simulink model "finalSimscapeModel"  (R2021b)
settings: Solver=FixedStepAuto  StartTime=0.0  StopTime=30+2*time_sequence(end)  FixedStep=0.05  RelTol=1e-3
libraries: nesl_utility x25, sm_lib x16, vrlib x6
settings Model: Creator=mukes  LastModifiedBy=mukes
settings ExplorerConfigSet: InternalSimMechanicsExplorerSettings="<ExplorerConfiguration><canonicalview>default</canonicalview><AnimationSetting><BasePlaybackSpeed>1.0</BasePlaybackSpeed><PlaybackSpeedFactor>1.0</PlaybackSpeedFactor></AnimationSetting><TilePanel><TileInfo><Tiles Columns=\"1\" Count=\"1\" Rows=\"1\"><Column Weight=\"1\"/><Row Weight=\"1\"/><Tile Height=\"1\" Width=\"1\" X=\"0\" Y=\"0\"/></Tiles></TileInfo><SceneInfo><SceneViewer><BGColor><R>0.60000002384185791</R><G>0.60000002384185791</G><B>0.60000002384185791</B></BGColor><Camera><DoPerspective>on</DoPerspective><Position><X>0.947420253079612085</X><Y>-0.0616353411456797562</Y><Z>0.809347594742444554</Z></Position><Center><X>-2.25255068230077837</X><Y>-0.872881532072153465</Y><Z>0.964544977754672184</Z></Center><Up><X>0.118811010900315428</X><Y>-0.286795567538067564</Y><Z>0.950595732227618839</Z></Up><ViewLimDist>1</ViewLimDist><YLim>0.466307658154998583</YLim><XLim>0.755157212465178973</XLim></Camera></SceneViewer></SceneInfo></TilePanel><MechEditorPanel><Cameras><Camera><Id>Camera1</Id><Value><Name>Camera1</Name><NativeCamera><PositionKeyframeSet><Keyframe><Time>50</Time><Value><X>2.03308088006994</X><Y>0.9365322772522765</Y><Z>2.5154667404724962</Z></Value></Keyframe></PositionKeyframeSet><CenterKeyframeSet><Keyframe><Time>50</Time><Value><X>-0.070008809160188701</X><Y>-0.63944287284674839</Y><Z>1.2349132743696094</Z></Value></Keyframe></CenterKeyframeSet><UpVectorKeyframeSet><Keyframe><Time>50</Time><Value><X>-0.43034741458034742</X><Y>-0.14909651685273262</Y><Z>0.89026475355727386</Z></Value></Keyframe></UpVectorKeyframeSet></NativeCamera></Value></Camera></Cameras><GfxPanelCameraMap><MapElement CameraMLId=\"Camera1\" GfxPanelIndex=\"0\"/></GfxPanelCameraMap><VideoCreator><PlaybackSpeedRatio>1.0</PlaybackSpeedRatio><FrameRate>30</FrameRate><VideoFormat>Motion JPEG AVI</VideoFormat><FrameSize>auto</FrameSize></VideoCreator></MechEditorPanel></ExplorerConfiguration>"

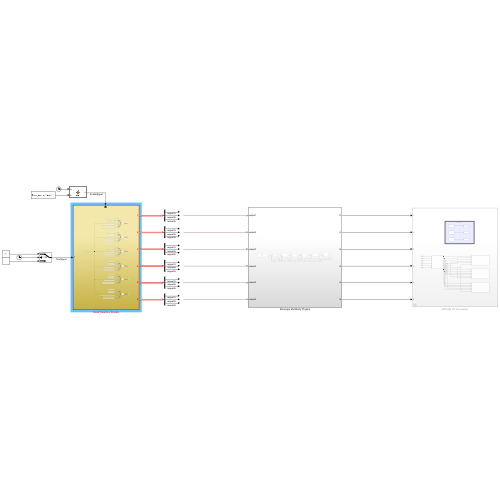
[thumbnail: Simulink's stored preview of the top-level diagram]
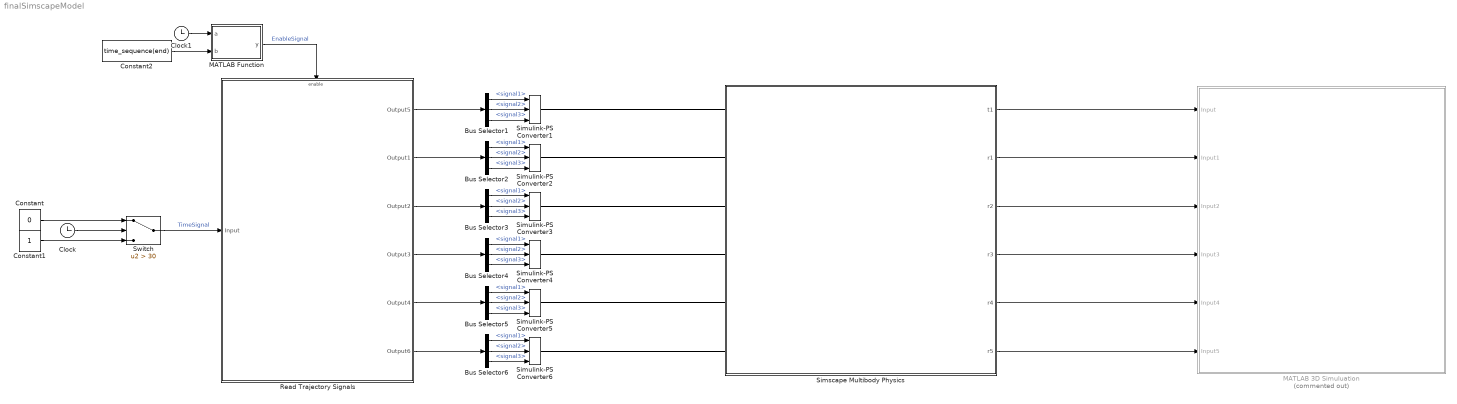
== system finalSimscapeModel ==
  Bus Selector{1..6} (6 alike) : BusSelector  OutputSignals=signal1,signal2,signal3
  Clock : Clock
  Clock1 : Clock
  Constant : Constant  Value=0
  Constant1 : Constant
  Constant2 : Constant  Value=time_sequence(end)
  MATLAB 3D Simuluation : Subsystem  Commented=on
  MATLAB Function : MATLAB Function  TreatAsAtomicUnit=on
  Read Trajectory Signals : Subsystem
  Simscape Multibody Physics : Subsystem
  Simulink-PS Converter{1..6} (6 alike) : nesl_utility/Simulink-PS Converter  PhysicalDomain=network_engine_domain  SubClassName=ps_input  LeftPortType=input  RightPortType=output  PseudoPeriodic=off  Frequencies=[]  NoiseDistribution=none  NoiseParameters=[]  Unit=1  AffineConversion=off  FilteringAndDerivatives=provide  SimscapeFilterOrder=1  InputFilterTimeConstant=0.001  UdotUserProvided=2
      settings: SourceProductBaseCode=PW,SS
  Switch : Switch  Criteria=u2 > Threshold  Threshold=30
  wires:
  Switch/1 -> Read Trajectory Signals/1(Input)  "TimeSignal"
  Constant/1 -> Switch/1
  Clock/1 -> Switch/2
  Constant1/1 -> Switch/3
  Bus Selector1/2 -> Simulink-PS Converter1/2  "<signal2>"
  Read Trajectory Signals/1(Output5) -> Bus Selector1/1
  Bus Selector1/3 -> Simulink-PS Converter1/3  "<signal3>"
  Bus Selector1/1 -> Simulink-PS Converter1/1  "<signal1>"
  Bus Selector2/2 -> Simulink-PS Converter2/2  "<signal2>"
  Read Trajectory Signals/2(Output1) -> Bus Selector2/1
  Bus Selector2/3 -> Simulink-PS Converter2/3  "<signal3>"
  Bus Selector2/1 -> Simulink-PS Converter2/1  "<signal1>"
  Bus Selector3/2 -> Simulink-PS Converter3/2  "<signal2>"
  Bus Selector3/1 -> Simulink-PS Converter3/1  "<signal1>"
  Bus Selector3/3 -> Simulink-PS Converter3/3  "<signal3>"
  Read Trajectory Signals/3(Output2) -> Bus Selector3/1
  Bus Selector4/2 -> Simulink-PS Converter4/2  "<signal2>"
  Bus Selector4/1 -> Simulink-PS Converter4/1  "<signal1>"
  Bus Selector4/3 -> Simulink-PS Converter4/3  "<signal3>"
  Read Trajectory Signals/4(Output3) -> Bus Selector4/1
  Bus Selector5/2 -> Simulink-PS Converter5/2  "<signal2>"
  Bus Selector5/1 -> Simulink-PS Converter5/1  "<signal1>"
  Bus Selector5/3 -> Simulink-PS Converter5/3  "<signal3>"
  Read Trajectory Signals/5(Output4) -> Bus Selector5/1
  Bus Selector6/2 -> Simulink-PS Converter6/2  "<signal2>"
  Bus Selector6/1 -> Simulink-PS Converter6/1  "<signal1>"
  Bus Selector6/3 -> Simulink-PS Converter6/3  "<signal3>"
  Read Trajectory Signals/6(Output6) -> Bus Selector6/1
  Clock1/1 -> MATLAB Function/1(a)
  Constant2/1 -> MATLAB Function/2(b)
  MATLAB Function/1(y) -> Read Trajectory Signals/Enable  "EnableSignal"
  Simscape Multibody Physics/1(t1) -> MATLAB 3D Simuluation/1(Input)
  Simscape Multibody Physics/2(r1) -> MATLAB 3D Simuluation/2(Input1)
  Simscape Multibody Physics/3(r2) -> MATLAB 3D Simuluation/3(Input2)
  Simscape Multibody Physics/4(r3) -> MATLAB 3D Simuluation/4(Input3)
  Simscape Multibody Physics/5(r4) -> MATLAB 3D Simuluation/5(Input4)
  Simscape Multibody Physics/6(r5) -> MATLAB 3D Simuluation/6(Input5)
  connections:
  Simulink-PS Converter1/RConn1 -- Simscape Multibody Physics/LConn1
  Simulink-PS Converter2/RConn1 -- Simscape Multibody Physics/LConn2
  Simulink-PS Converter3/RConn1 -- Simscape Multibody Physics/LConn3
  Simulink-PS Converter4/RConn1 -- Simscape Multibody Physics/LConn4
  Simulink-PS Converter5/RConn1 -- Simscape Multibody Physics/LConn5
  Simulink-PS Converter6/RConn1 -- Simscape Multibody Physics/LConn6

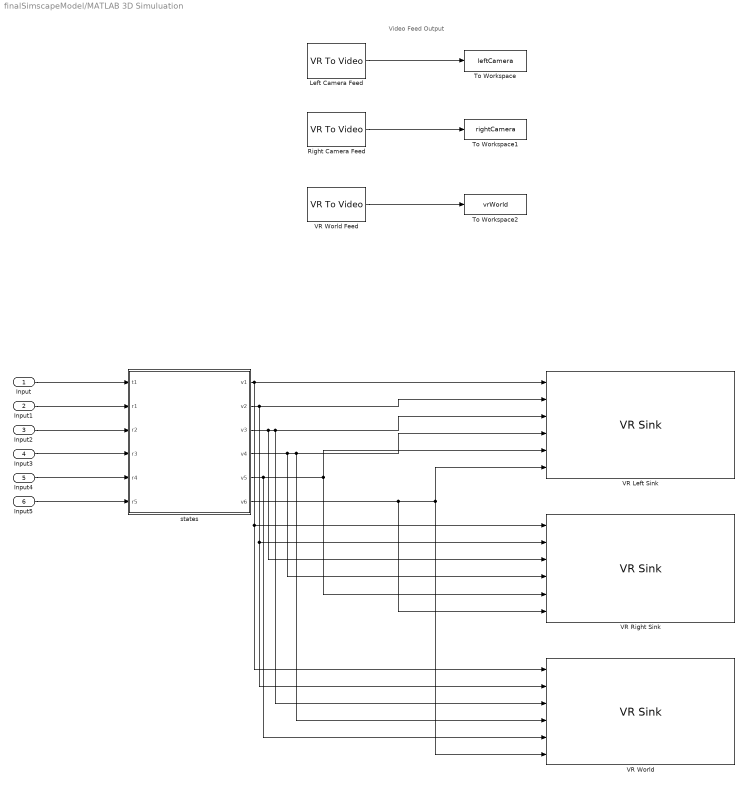
== system finalSimscapeModel/MATLAB 3D Simuluation ==
  note: Video Feed Output
  Input : Inport
  Input1 : Inport  Port=2
  Input2 : Inport  Port=3
  Input3 : Inport  Port=4
  Input4 : Inport  Port=5
  Input5 : Inport  Port=6
  Left Camera Feed : vrlib/VR To Video  InstantiateOnLoad=on  SampleTime=0.1  ViewEnable=on  RemoteChange=off  RemoteView=off  WorldFileName=jlr_world_final2_left.x3d  WorldDescription=Straight Road Strip - 2 Lanes  AutoView=off  VideoDimensions=[1080 1920]  AllowVariableSize=off
      settings: SourceProductBaseCode=SL
  Right Camera Feed : vrlib/VR To Video  InstantiateOnLoad=on  SampleTime=0.1  ViewEnable=on  RemoteChange=off  RemoteView=off  WorldFileName=jlr_world_final2_right.x3d  WorldDescription=Straight Road Strip - 2 Lanes  AutoView=off  VideoDimensions=[1080 1920]  AllowVariableSize=off
      settings: SourceProductBaseCode=SL
  To Workspace : ToWorkspace  VariableName=leftCamera  SaveFormat=Timeseries  SampleTime=-1
  To Workspace1 : ToWorkspace  VariableName=rightCamera  SaveFormat=Timeseries  SampleTime=-1
  To Workspace2 : ToWorkspace  VariableName=vrWorld  SaveFormat=Timeseries  SampleTime=-1
  VR Left Sink : vrlib/VR Sink  InstantiateOnLoad=on  SampleTime=0.1  ViewEnable=on  RemoteChange=off  RemoteView=off  FieldsWritten=axis_Trans1.translation.3.1.1.double#axis_Rev1.rotation.4.1.1.double#axis_Rev2.rotation.4.1.1.double#axis_Rev3.rotation.4.1.1.double#axis_Rev4.rotation.4.1.1.double#axis_Rev5.rotation.4.1.1.double  WorldFileName=jlr_world_final2_left.x3d  WorldDescription=Straight Road Strip - 2 Lanes  AutoView=off  VideoDimensions=[]  AllowVariableSize=off
  VR Right Sink : vrlib/VR Sink  InstantiateOnLoad=on  SampleTime=0.1  ViewEnable=on  RemoteChange=off  RemoteView=off  FieldsWritten=axis_Trans1.translation.3.1.1.double#axis_Rev1.rotation.4.1.1.double#axis_Rev2.rotation.4.1.1.double#axis_Rev3.rotation.4.1.1.double#axis_Rev4.rotation.4.1.1.double#axis_Rev5.rotation.4.1.1.double  WorldFileName=jlr_world_final2_right.x3d  WorldDescription=Straight Road Strip - 2 Lanes  AutoView=off  VideoDimensions=[]  AllowVariableSize=off
  VR World : vrlib/VR Sink  InstantiateOnLoad=on  SampleTime=0.1  ViewEnable=on  RemoteChange=off  RemoteView=off  FieldsWritten=axis_Trans1.translation.3.1.1.double#axis_Rev1.rotation.4.1.1.double#axis_Rev2.rotation.4.1.1.double#axis_Rev3.rotation.4.1.1.double#axis_Rev4.rotation.4.1.1.double#axis_Rev5.rotation.4.1.1.double  WorldFileName=jlr_world_final2.x3d  WorldDescription=Straight Road Strip - 2 Lanes  AutoView=off  VideoDimensions=[]  AllowVariableSize=off
  VR World Feed : vrlib/VR To Video  InstantiateOnLoad=on  SampleTime=0.1  ViewEnable=on  RemoteChange=off  RemoteView=off  WorldFileName=jlr_world_final2.x3d  WorldDescription=Straight Road Strip - 2 Lanes  AutoView=off  VideoDimensions=[1080 1920]  AllowVariableSize=off
      settings: SourceProductBaseCode=SL
  states : MATLAB Function  TreatAsAtomicUnit=on
  wires:
  states/6(v6) -> VR World/6, VR Left Sink/6, VR Right Sink/6
  states/5(v5) -> VR Right Sink/5, VR Left Sink/5, VR World/5
  states/4(v4) -> VR World/4, VR Left Sink/4, VR Right Sink/4
  states/1(v1) -> VR Right Sink/1, VR World/1, VR Left Sink/1
  states/2(v2) -> VR World/2, VR Right Sink/2, VR Left Sink/2
  Input2/1 -> states/3(r2)
  states/3(v3) -> VR World/3, VR Left Sink/3, VR Right Sink/3
  Input4/1 -> states/5(r4)
  Input1/1 -> states/2(r1)
  Input5/1 -> states/6(r5)
  Input3/1 -> states/4(r3)
  Input/1 -> states/1(t1)
  Left Camera Feed/1 -> To Workspace/1
  Right Camera Feed/1 -> To Workspace1/1
  VR World Feed/1 -> To Workspace2/1

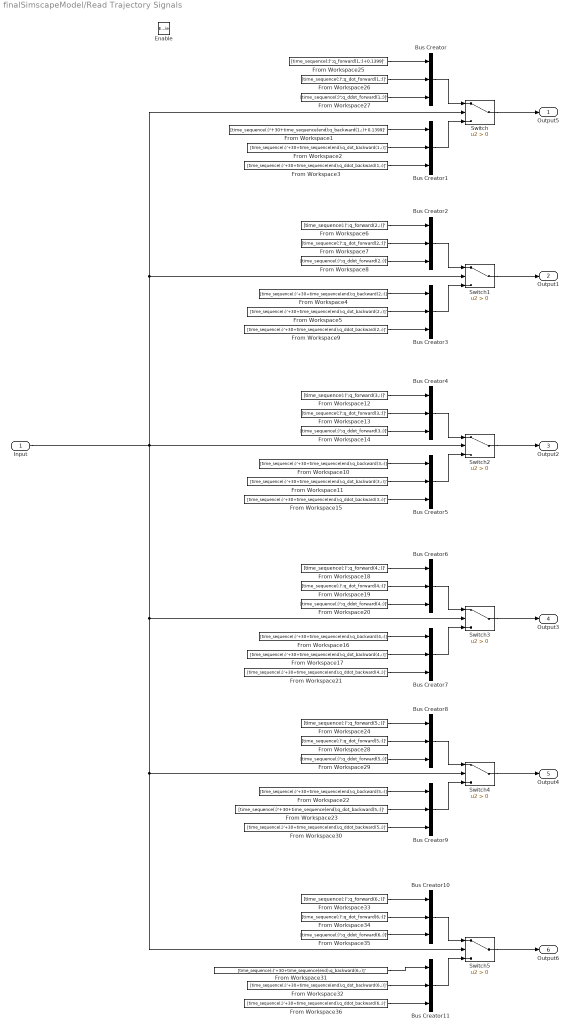
== system finalSimscapeModel/Read Trajectory Signals ==
  Input : Inport
  Enable : EnablePort
  Bus Creator{,1..11} (12 alike) : BusCreator  Inputs=3
  From Workspace1 : FromWorkspace  VariableName=[time_sequence(:)'+30+time_sequence(end);q_backward(1,:)+0.1399]'
  From Workspace10 : FromWorkspace  VariableName=[time_sequence(:)'+30+time_sequence(end);q_backward(3,:)]'
  From Workspace11 : FromWorkspace  VariableName=[time_sequence(:)'+30+time_sequence(end);q_dot_backward(3,:)]'
  From Workspace12 : FromWorkspace  VariableName=[time_sequence(:)';q_forward(3,:)]'
  From Workspace13 : FromWorkspace  VariableName=[time_sequence(:)';q_dot_forward(3,:)]'
  From Workspace14 : FromWorkspace  VariableName=[time_sequence(:)';q_ddot_forward(3,:)]'
  From Workspace15 : FromWorkspace  VariableName=[time_sequence(:)'+30+time_sequence(end);q_ddot_backward(3,:)]'
  From Workspace16 : FromWorkspace  VariableName=[time_sequence(:)'+30+time_sequence(end);q_backward(4,:)]'
  From Workspace17 : FromWorkspace  VariableName=[time_sequence(:)'+30+time_sequence(end);q_dot_backward(4,:)]'
  From Workspace18 : FromWorkspace  VariableName=[time_sequence(:)';q_forward(4,:)]'
  From Workspace19 : FromWorkspace  VariableName=[time_sequence(:)';q_dot_forward(4,:)]'
  From Workspace2 : FromWorkspace  VariableName=[time_sequence(:)'+30+time_sequence(end);q_dot_backward(1,:)]'
  From Workspace20 : FromWorkspace  VariableName=[time_sequence(:)';q_ddot_forward(4,:)]'
  From Workspace21 : FromWorkspace  VariableName=[time_sequence(:)'+30+time_sequence(end);q_ddot_backward(4,:)]'
  From Workspace22 : FromWorkspace  VariableName=[time_sequence(:)'+30+time_sequence(end);q_backward(5,:)]'
  From Workspace23 : FromWorkspace  VariableName=[time_sequence(:)'+30+time_sequence(end);q_dot_backward(5,:)]'
  From Workspace24 : FromWorkspace  VariableName=[time_sequence(:)';q_forward(5,:)]'
  From Workspace25 : FromWorkspace  VariableName=[time_sequence(:)';q_forward(1,:)+0.1399]'
  From Workspace26 : FromWorkspace  VariableName=[time_sequence(:)';q_dot_forward(1,:)]'
  From Workspace27 : FromWorkspace  VariableName=[time_sequence(:)';q_ddot_forward(1,:)]'
  From Workspace28 : FromWorkspace  VariableName=[time_sequence(:)';q_dot_forward(5,:)]'
  From Workspace29 : FromWorkspace  VariableName=[time_sequence(:)';q_ddot_forward(5,:)]'
  From Workspace3 : FromWorkspace  VariableName=[time_sequence(:)'+30+time_sequence(end);q_ddot_backward(1,:)]'
  From Workspace30 : FromWorkspace  VariableName=[time_sequence(:)'+30+time_sequence(end);q_ddot_backward(5,:)]'
  From Workspace31 : FromWorkspace  VariableName=[time_sequence(:)'+30+time_sequence(end);q_backward(6,:)]'
  From Workspace32 : FromWorkspace  VariableName=[time_sequence(:)'+30+time_sequence(end);q_dot_backward(6,:)]'
  From Workspace33 : FromWorkspace  VariableName=[time_sequence(:)';q_forward(6,:)]'
  From Workspace34 : FromWorkspace  VariableName=[time_sequence(:)';q_dot_forward(6,:)]'
  From Workspace35 : FromWorkspace  VariableName=[time_sequence(:)';q_ddot_forward(6,:)]'
  From Workspace36 : FromWorkspace  VariableName=[time_sequence(:)'+30+time_sequence(end);q_ddot_backward(6,:)]'
  From Workspace4 : FromWorkspace  VariableName=[time_sequence(:)'+30+time_sequence(end);q_backward(2,:)]'
  From Workspace5 : FromWorkspace  VariableName=[time_sequence(:)'+30+time_sequence(end);q_dot_backward(2,:)]'
  From Workspace6 : FromWorkspace  VariableName=[time_sequence(:)';q_forward(2,:)]'
  From Workspace7 : FromWorkspace  VariableName=[time_sequence(:)';q_dot_forward(2,:)]'
  From Workspace8 : FromWorkspace  VariableName=[time_sequence(:)';q_ddot_forward(2,:)]'
  From Workspace9 : FromWorkspace  VariableName=[time_sequence(:)'+30+time_sequence(end);q_ddot_backward(2,:)]'
  Switch{,1..5} (6 alike) : Switch  Criteria=u2 > Threshold
  Output5 : Outport
  Output1 : Outport  Port=2
  Output2 : Outport  Port=3
  Output3 : Outport  Port=4
  Output4 : Outport  Port=5
  Output6 : Outport  Port=6
  wires:
  From Workspace25/1 -> Bus Creator/1
  From Workspace26/1 -> Bus Creator/2
  From Workspace27/1 -> Bus Creator/3
  From Workspace1/1 -> Bus Creator1/1
  From Workspace3/1 -> Bus Creator1/3
  From Workspace2/1 -> Bus Creator1/2
  Bus Creator/1 -> Switch/1
  Bus Creator1/1 -> Switch/3
  Input/1 -> Switch1/2, Switch/2, Switch2/2, Switch5/2, Switch4/2, Switch3/2
  Switch/1 -> Output5/1
  Switch1/1 -> Output1/1
  From Workspace4/1 -> Bus Creator3/1
  Bus Creator3/1 -> Switch1/3
  From Workspace6/1 -> Bus Creator2/1
  From Workspace7/1 -> Bus Creator2/2
  Bus Creator2/1 -> Switch1/1
  From Workspace9/1 -> Bus Creator3/3
  From Workspace5/1 -> Bus Creator3/2
  From Workspace8/1 -> Bus Creator2/3
  Switch2/1 -> Output2/1
  From Workspace10/1 -> Bus Creator5/1
  Bus Creator5/1 -> Switch2/3
  From Workspace12/1 -> Bus Creator4/1
  From Workspace13/1 -> Bus Creator4/2
  Bus Creator4/1 -> Switch2/1
  From Workspace15/1 -> Bus Creator5/3
  From Workspace11/1 -> Bus Creator5/2
  From Workspace14/1 -> Bus Creator4/3
  Switch3/1 -> Output3/1
  From Workspace16/1 -> Bus Creator7/1
  Bus Creator7/1 -> Switch3/3
  From Workspace18/1 -> Bus Creator6/1
  From Workspace19/1 -> Bus Creator6/2
  Bus Creator6/1 -> Switch3/1
  From Workspace21/1 -> Bus Creator7/3
  From Workspace17/1 -> Bus Creator7/2
  From Workspace20/1 -> Bus Creator6/3
  Switch4/1 -> Output4/1
  From Workspace22/1 -> Bus Creator9/1
  Bus Creator9/1 -> Switch4/3
  From Workspace24/1 -> Bus Creator8/1
  From Workspace28/1 -> Bus Creator8/2
  Bus Creator8/1 -> Switch4/1
  From Workspace30/1 -> Bus Creator9/3
  From Workspace23/1 -> Bus Creator9/2
  From Workspace29/1 -> Bus Creator8/3
  Switch5/1 -> Output6/1
  From Workspace31/1 -> Bus Creator11/1
  Bus Creator11/1 -> Switch5/3
  From Workspace33/1 -> Bus Creator10/1
  From Workspace34/1 -> Bus Creator10/2
  Bus Creator10/1 -> Switch5/1
  From Workspace36/1 -> Bus Creator11/3
  From Workspace32/1 -> Bus Creator11/2
  From Workspace35/1 -> Bus Creator10/3

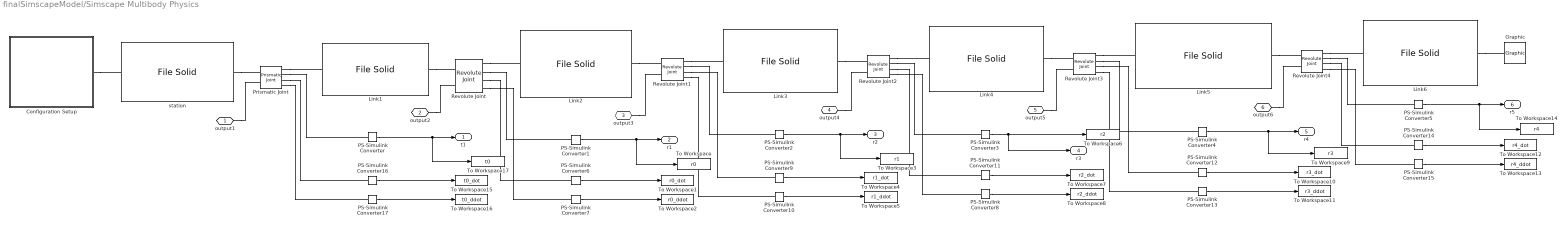
== system finalSimscapeModel/Simscape Multibody Physics ==
  Configuration Setup : Subsystem
  Graphic : sm_lib/Body Elements/Graphic  GraphicType=Marker  MarkerShape=Sphere  MarkerSize=10  GraphicVisPropType=SimpleVisualProperties  GraphicDiffuseColor=[1 0 0]  GraphicSpecularColor=[0.5 0.5 0.5 1.0]  GraphicAmbientColor=[0.15 0.15 0.15 1.0]  GraphicEmissiveColor=[0.0 0.0 0.0 1.0]  GraphicShininess=75  GraphicOpacity=1.0
  Link1 : sm_lib/Body Elements/File Solid  ExtGeomFileName=C:\Users\mukes\Downloads\Robot-Arm\Simscape Simulation\cadModels\Link1.STEP  UnitType=FromFile  ExtGeomFileUnits=m  StepReaderType=HEX  ExportConvexHullGeometry=off  InertiaType=CalculateFromGeometry  Mass=1  MassUnits=kg  CenterOfMass=[0 0 0]  CenterOfMassUnits=m  MomentsOfInertia=[1 1 1]  MomentsOfInertiaUnits=kg*m^2  ProductsOfInertia=[0 0 0]  ProductsOfInertiaUnits=kg*m^2  BasedOnType=Density  Density=1000  DensityUnits=kg/m^3  DoExposeReferenceFrame=off  SerializedFrames=<Frames><Frame><Id>Frame1</Id><Value><Name>prismaticJoint</Name><Origin><Source>GeometricFeature</Source><FeatureName>circular curve 1514</FeatureName></Origin><PrimaryAxis><DefinedDirection>+Z</DefinedDirection><Source>GeometricFeature</Source><SourceDirection>+Z</SourceDirection><FeatureName>circular curve 1514</FeatureName></PrimaryAxis><SecondaryAxis><DefinedDirection>+X</DefinedDirection><Source>GeometricFeature</Source><SourceDirection>+X</SourceDirection><FeatureName>segment 1580</FeatureName></SecondaryAxis></Value></Frame><Frame><Id>Frame2</Id><Value><Name>revoluteJoint</Name><Origin><Source>GeometricFeature</Source><FeatureName>circular curve 835</FeatureName></Origin><PrimaryAxis><DefinedDirection>-Z</DefinedDirection><Source>GeometricFeature</Source><SourceDirection>+Z</SourceDirection><FeatureName>circular curve 835</FeatureName></PrimaryAxis><SecondaryAxis><DefinedDirection>+X</DefinedDirection><Source>GeometricFeature</Source><SourceDirection>+X</SourceDirection><FeatureName>segment 1054</FeatureName></SecondaryAxis></Value></Frame></Frames>  GraphicType=FromGeometry  MarkerShape=Sphere  MarkerSize=10  GraphicVisPropType=SimpleVisualProperties  GraphicDiffuseColor=[0.5 0.5 0.5]  GraphicSpecularColor=[0.5 0.5 0.5 1.0]  GraphicAmbientColor=[0.15 0.15 0.15 1.0]  GraphicEmissiveColor=[0.0 0.0 0.0 1.0]  GraphicShininess=75  GraphicOpacity=1.0
  Link2 : sm_lib/Body Elements/File Solid  ExtGeomFileName=.\cadModels\Link2.STEP  UnitType=FromFile  ExtGeomFileUnits=m  StepReaderType=HEX  ExportConvexHullGeometry=off  InertiaType=CalculateFromGeometry  Mass=1  MassUnits=kg  CenterOfMass=[0 0 0]  CenterOfMassUnits=m  MomentsOfInertia=[1 1 1]  MomentsOfInertiaUnits=kg*m^2  ProductsOfInertia=[0 0 0]  ProductsOfInertiaUnits=kg*m^2  BasedOnType=Density  Density=1000  DensityUnits=kg/m^3  DoExposeReferenceFrame=off  SerializedFrames=<Frames><Frame><Id>Frame1</Id><Value><Name>revoluteJoint1</Name><Origin><Source>GeometricFeature</Source><FeatureName>circular curve 1127</FeatureName></Origin><PrimaryAxis><DefinedDirection>-Z</DefinedDirection><Source>GeometricFeature</Source><SourceDirection>+Z</SourceDirection><FeatureName>circular curve 1129</FeatureName></PrimaryAxis><SecondaryAxis><DefinedDirection>+Y</DefinedDirection><Source>GeometricFeature</Source><SourceDirection>+X</SourceDirection><FeatureName>segment 1270</FeatureName></SecondaryAxis></Value></Frame><Frame><Id>Frame2</Id><Value><Name>revoluteJoint2</Name><Origin><Source>GeometricFeature</Source><FeatureName>circular curve 892</FeatureName></Origin><PrimaryAxis><DefinedDirection>-Z</DefinedDirection><Source>GeometricFeature</Source><SourceDirection>+Z</SourceDirection><FeatureName>circular curve 893</FeatureName></PrimaryAxis><SecondaryAxis><DefinedDirection>+Y</DefinedDirection><Source>ReferenceFrame</Source><SourceDirection>+X</SourceDirection><FeatureName></FeatureName></SecondaryAxis></Value></Frame></Frames>  GraphicType=FromGeometry  MarkerShape=Sphere  MarkerSize=10  GraphicVisPropType=SimpleVisualProperties  GraphicDiffuseColor=[0.5 0.5 0.5]  GraphicSpecularColor=[0.5 0.5 0.5 1.0]  GraphicAmbientColor=[0.15 0.15 0.15 1.0]  GraphicEmissiveColor=[0.0 0.0 0.0 1.0]  GraphicShininess=75  GraphicOpacity=1.0
  Link3 : sm_lib/Body Elements/File Solid  ExtGeomFileName=.\cadModels\Link3.STEP  UnitType=FromFile  ExtGeomFileUnits=m  StepReaderType=HEX  ExportConvexHullGeometry=off  InertiaType=CalculateFromGeometry  Mass=1  MassUnits=kg  CenterOfMass=[0 0 0]  CenterOfMassUnits=m  MomentsOfInertia=[1 1 1]  MomentsOfInertiaUnits=kg*m^2  ProductsOfInertia=[0 0 0]  ProductsOfInertiaUnits=kg*m^2  BasedOnType=Density  Density=1000  DensityUnits=kg/m^3  DoExposeReferenceFrame=off  SerializedFrames=<Frames><Frame><Id>Frame1</Id><Value><Name>revoluteJoint2</Name><Origin><Source>GeometricFeature</Source><FeatureName>circular curve 65</FeatureName></Origin><PrimaryAxis><DefinedDirection>-Z</DefinedDirection><Source>GeometricFeature</Source><SourceDirection>+Z</SourceDirection><FeatureName>circular curve 65</FeatureName></PrimaryAxis><SecondaryAxis><DefinedDirection>-Y</DefinedDirection><Source>GeometricFeature</Source><SourceDirection>+X</SourceDirection><FeatureName>segment 47</FeatureName></SecondaryAxis></Value></Frame><Frame><Id>Frame2</Id><Value><Name>revoluteJoint3</Name><Origin><Source>GeometricFeature</Source><FeatureName>circular curve 10</FeatureName></Origin><PrimaryAxis><DefinedDirection>+Z</DefinedDirection><Source>GeometricFeature</Source><SourceDirection>+Z</SourceDirection><FeatureName>circular curve 10</FeatureName></PrimaryAxis><SecondaryAxis><DefinedDirection>+X</DefinedDirection><Source>ReferenceFrame</Source><SourceDirection>+X</SourceDirection><FeatureName></FeatureName></SecondaryAxis></Value></Frame></Frames>  GraphicType=FromGeometry  MarkerShape=Sphere  MarkerSize=10  GraphicVisPropType=SimpleVisualProperties  GraphicDiffuseColor=[0.5 0.5 0.5]  GraphicSpecularColor=[0.5 0.5 0.5 1.0]  GraphicAmbientColor=[0.15 0.15 0.15 1.0]  GraphicEmissiveColor=[0.0 0.0 0.0 1.0]  GraphicShininess=75  GraphicOpacity=1.0
  Link4 : sm_lib/Body Elements/File Solid  ExtGeomFileName=.\cadModels\Link4.STEP  UnitType=FromFile  ExtGeomFileUnits=m  StepReaderType=HEX  ExportConvexHullGeometry=off  InertiaType=CalculateFromGeometry  Mass=1  MassUnits=kg  CenterOfMass=[0 0 0]  CenterOfMassUnits=m  MomentsOfInertia=[1 1 1]  MomentsOfInertiaUnits=kg*m^2  ProductsOfInertia=[0 0 0]  ProductsOfInertiaUnits=kg*m^2  BasedOnType=Density  Density=1000  DensityUnits=kg/m^3  DoExposeReferenceFrame=off  SerializedFrames=<Frames><Frame><Id>Frame1</Id><Value><Name>revoluteJoint3</Name><Origin><Source>GeometricFeature</Source><FeatureName>circular curve 254</FeatureName></Origin><PrimaryAxis><DefinedDirection>+Z</DefinedDirection><Source>GeometricFeature</Source><SourceDirection>+Z</SourceDirection><FeatureName>circular curve 250</FeatureName></PrimaryAxis><SecondaryAxis><DefinedDirection>-X</DefinedDirection><Source>GeometricFeature</Source><SourceDirection>+X</SourceDirection><FeatureName>segment 125</FeatureName></SecondaryAxis></Value></Frame><Frame><Id>Frame2</Id><Value><Name>revoluteJoint4</Name><Origin><Source>GeometricFeature</Source><FeatureName>circular curve 319</FeatureName></Origin><PrimaryAxis><DefinedDirection>+Z</DefinedDirection><Source>GeometricFeature</Source><SourceDirection>+Z</SourceDirection><FeatureName>circular curve 319</FeatureName></PrimaryAxis><SecondaryAxis><DefinedDirection>+X</DefinedDirection><Source>ReferenceFrame</Source><SourceDirection>+X</SourceDirection><FeatureName></FeatureName></SecondaryAxis></Value></Frame></Frames>  GraphicType=FromGeometry  MarkerShape=Sphere  MarkerSize=10  GraphicVisPropType=SimpleVisualProperties  GraphicDiffuseColor=[0.5 0.5 0.5]  GraphicSpecularColor=[0.5 0.5 0.5 1.0]  GraphicAmbientColor=[0.15 0.15 0.15 1.0]  GraphicEmissiveColor=[0.0 0.0 0.0 1.0]  GraphicShininess=75  GraphicOpacity=1.0
  Link5 : sm_lib/Body Elements/File Solid  ExtGeomFileName=.\cadModels\Link5.STEP  UnitType=FromFile  ExtGeomFileUnits=m  StepReaderType=HEX  ExportConvexHullGeometry=off  InertiaType=CalculateFromGeometry  Mass=1  MassUnits=kg  CenterOfMass=[0 0 0]  CenterOfMassUnits=m  MomentsOfInertia=[1 1 1]  MomentsOfInertiaUnits=kg*m^2  ProductsOfInertia=[0 0 0]  ProductsOfInertiaUnits=kg*m^2  BasedOnType=Density  Density=1000  DensityUnits=kg/m^3  DoExposeReferenceFrame=off  SerializedFrames=<Frames><Frame><Id>Frame1</Id><Value><Name>revoluteJoint4</Name><Origin><Source>GeometricFeature</Source><FeatureName>circular curve 94</FeatureName></Origin><PrimaryAxis><DefinedDirection>-Z</DefinedDirection><Source>GeometricFeature</Source><SourceDirection>+Z</SourceDirection><FeatureName>circular curve 94</FeatureName></PrimaryAxis><SecondaryAxis><DefinedDirection>+X</DefinedDirection><Source>GeometricFeature</Source><SourceDirection>+X</SourceDirection><FeatureName>segment 289</FeatureName></SecondaryAxis></Value></Frame><Frame><Id>Frame2</Id><Value><Name>revoluteJoint5</Name><Origin><Source>GeometricFeature</Source><FeatureName>circular curve 36</FeatureName></Origin><PrimaryAxis><DefinedDirection>-Z</DefinedDirection><Source>GeometricFeature</Source><SourceDirection>+Z</SourceDirection><FeatureName>circular curve 36</FeatureName></PrimaryAxis><SecondaryAxis><DefinedDirection>-X</DefinedDirection><Source>GeometricFeature</Source><SourceDirection>+X</SourceDirection><FeatureName>segment 73</FeatureName></SecondaryAxis></Value></Frame></Frames>  GraphicType=FromGeometry  MarkerShape=Sphere  MarkerSize=10  GraphicVisPropType=SimpleVisualProperties  GraphicDiffuseColor=[0.5 0.5 0.5]  GraphicSpecularColor=[0.5 0.5 0.5 1.0]  GraphicAmbientColor=[0.15 0.15 0.15 1.0]  GraphicEmissiveColor=[0.0 0.0 0.0 1.0]  GraphicShininess=75  GraphicOpacity=1.0
  Link6 : sm_lib/Body Elements/File Solid  ExtGeomFileName=.\cadModels\end_effector.STEP  UnitType=FromFile  ExtGeomFileUnits=m  StepReaderType=HEX  ExportConvexHullGeometry=off  InertiaType=PointMass  Mass=1  MassUnits=kg  CenterOfMass=[0 0 0]  CenterOfMassUnits=m  MomentsOfInertia=[1 1 1]  MomentsOfInertiaUnits=kg*m^2  ProductsOfInertia=[0 0 0]  ProductsOfInertiaUnits=kg*m^2  BasedOnType=Density  Density=1000  DensityUnits=kg/m^3  DoExposeReferenceFrame=off  SerializedFrames=<Frames><Frame><Id>Frame1</Id><Value><Name>revoluteJoint5</Name><Origin><Source>GeometricFeature</Source><FeatureName>circular curve 459</FeatureName></Origin><PrimaryAxis><DefinedDirection>-Z</DefinedDirection><Source>GeometricFeature</Source><SourceDirection>+Z</SourceDirection><FeatureName>circular curve 341</FeatureName></PrimaryAxis><SecondaryAxis><DefinedDirection>+X</DefinedDirection><Source>GeometricFeature</Source><SourceDirection>+X</SourceDirection><FeatureName>segment 552</FeatureName></SecondaryAxis></Value></Frame><Frame><Id>Frame2</Id><Value><Name>finalMarker</Name><Origin><Source>GeometricFeature</Source><FeatureName>circular curve 161</FeatureName></Origin><PrimaryAxis><DefinedDirection>+Z</DefinedDirection><Source>GeometricFeature</Source><SourceDirection>+Z</SourceDirection><FeatureName>circular curve 161</FeatureName></PrimaryAxis><SecondaryAxis><DefinedDirection>+X</DefinedDirection><Source>ReferenceFrame</Source><SourceDirection>+Y</SourceDirection><FeatureName></FeatureName></SecondaryAxis></Value></Frame></Frames>  GraphicType=FromGeometry  MarkerShape=Sphere  MarkerSize=10  GraphicVisPropType=SimpleVisualProperties  GraphicDiffuseColor=[0.5 0.5 0.5]  GraphicSpecularColor=[0.5 0.5 0.5 1.0]  GraphicAmbientColor=[0.15 0.15 0.15 1.0]  GraphicEmissiveColor=[0.0 0.0 0.0 1.0]  GraphicShininess=75  GraphicOpacity=1.0
  PS-Simulink Converter{,1..17} (18 alike) : nesl_utility/PS-Simulink Converter  PhysicalDomain=network_engine_domain  SubClassName=ps_output  LeftPortType=input  RightPortType=output  PseudoPeriodic=off  Frequencies=[]  Unit=inherit  AffineConversion=off
      settings: SourceProductBaseCode=PW,SS
  Prismatic Joint : sm_lib/Joints/Prismatic Joint  JointMode=Normal  SenseConstraintForce=off  SenseConstraintForceX=off  SenseConstraintForceY=off  SenseConstraintForceZ=off  SenseConstraintTorque=off  SenseConstraintTorqueX=off  SenseConstraintTorqueY=off  SenseConstraintTorqueZ=off  SenseTotalForce=off  SenseTotalForceX=off  SenseTotalForceY=off  SenseTotalForceZ=off  SenseTotalTorque=off  SenseTotalTorqueX=off  SenseTotalTorqueY=off  SenseTotalTorqueZ=off  CompositeWrenchDir=FollowerOnBase  CompositeWrenchFrame=BaseFrame  EquilibriumPosition=0  EquilibriumPositionUnits=m  SpringStiffness=0  SpringStiffnessUnits=N/m  DampingCoefficient=0  DampingCoefficientUnits=N/(m/s)  TorqueActuationMode=ComputedTorque  MotionActuationMode=InputMotion  SensePosition=on  SenseVelocity=on  SenseAcceleration=on  SenseTorqueForce=off  SenseLowerLimitTorqueForce=off  SenseUpperLimitTorqueForce=off  LowerLimitSpecify=off  LowerLimitBound=-1  LowerLimitBoundUnits=m  LowerLimitStiffness=1e6  LowerLimitStiffnessUnits=N/m  LowerLimitDamping=1e3  LowerLimitDampingUnits=N/(m/s)  LowerLimitTransitionRegionWidth=1e-4  LowerLimitTransitionRegionWidthUnits=m  UpperLimitSpecify=off  UpperLimitBound=1  UpperLimitBoundUnits=m  UpperLimitStiffness=1e6  UpperLimitStiffnessUnits=N/m  UpperLimitDamping=1e3  UpperLimitDampingUnits=N/(m/s)  UpperLimitTransitionRegionWidth=1e-4  UpperLimitTransitionRegionWidthUnits=m  PositionTargetSpecify=off  PositionTargetPriority=High  PositionTargetValue=0  PositionTargetValueUnits=m  VelocityTargetSpecify=off  VelocityTargetPriority=High  VelocityTargetValue=0  VelocityTargetValueUnits=m/s
  Revolute Joint : sm_lib/Joints/Revolute Joint  JointMode=Normal  SenseConstraintForce=off  SenseConstraintForceX=off  SenseConstraintForceY=off  SenseConstraintForceZ=off  SenseConstraintTorque=off  SenseConstraintTorqueX=off  SenseConstraintTorqueY=off  SenseConstraintTorqueZ=off  SenseTotalForce=off  SenseTotalForceX=off  SenseTotalForceY=off  SenseTotalForceZ=off  SenseTotalTorque=off  SenseTotalTorqueX=off  SenseTotalTorqueY=off  SenseTotalTorqueZ=off  CompositeWrenchDir=FollowerOnBase  CompositeWrenchFrame=BaseFrame  EquilibriumPosition=0  EquilibriumPositionUnits=deg  SpringStiffness=0  SpringStiffnessUnits=N*m/deg  DampingCoefficient=0  DampingCoefficientUnits=N*m/(deg/s)  TorqueActuationMode=ComputedTorque  MotionActuationMode=InputMotion  SensePosition=on  SenseVelocity=on  SenseAcceleration=on  SenseTorqueForce=off  SenseLowerLimitTorqueForce=off  SenseUpperLimitTorqueForce=off  LowerLimitSpecify=off  LowerLimitBound=-90  LowerLimitBoundUnits=deg  LowerLimitStiffness=1e4  LowerLimitStiffnessUnits=N*m/deg  LowerLimitDamping=10  LowerLimitDampingUnits=N*m/(deg/s)  LowerLimitTransitionRegionWidth=0.1  LowerLimitTransitionRegionWidthUnits=deg  UpperLimitSpecify=off  UpperLimitBound=90  UpperLimitBoundUnits=deg  UpperLimitStiffness=1e4  UpperLimitStiffnessUnits=N*m/deg  UpperLimitDamping=10  UpperLimitDampingUnits=N*m/(deg/s)  UpperLimitTransitionRegionWidth=0.1  UpperLimitTransitionRegionWidthUnits=deg  PositionTargetSpecify=off  PositionTargetPriority=High  PositionTargetValue=0  PositionTargetValueUnits=deg  VelocityTargetSpecify=off  VelocityTargetPriority=High  VelocityTargetValue=0  VelocityTargetValueUnits=deg/s
  Revolute Joint1 : sm_lib/Joints/Revolute Joint  JointMode=Normal  SenseConstraintForce=off  SenseConstraintForceX=off  SenseConstraintForceY=off  SenseConstraintForceZ=off  SenseConstraintTorque=off  SenseConstraintTorqueX=off  SenseConstraintTorqueY=off  SenseConstraintTorqueZ=off  SenseTotalForce=off  SenseTotalForceX=off  SenseTotalForceY=off  SenseTotalForceZ=off  SenseTotalTorque=off  SenseTotalTorqueX=off  SenseTotalTorqueY=off  SenseTotalTorqueZ=off  CompositeWrenchDir=FollowerOnBase  CompositeWrenchFrame=BaseFrame  EquilibriumPosition=0  EquilibriumPositionUnits=deg  SpringStiffness=0  SpringStiffnessUnits=N*m/deg  DampingCoefficient=0  DampingCoefficientUnits=N*m/(deg/s)  TorqueActuationMode=ComputedTorque  MotionActuationMode=InputMotion  SensePosition=on  SenseVelocity=on  SenseAcceleration=on  SenseTorqueForce=off  SenseLowerLimitTorqueForce=off  SenseUpperLimitTorqueForce=off  LowerLimitSpecify=off  LowerLimitBound=-90  LowerLimitBoundUnits=deg  LowerLimitStiffness=1e4  LowerLimitStiffnessUnits=N*m/deg  LowerLimitDamping=10  LowerLimitDampingUnits=N*m/(deg/s)  LowerLimitTransitionRegionWidth=0.1  LowerLimitTransitionRegionWidthUnits=deg  UpperLimitSpecify=off  UpperLimitBound=90  UpperLimitBoundUnits=deg  UpperLimitStiffness=1e4  UpperLimitStiffnessUnits=N*m/deg  UpperLimitDamping=10  UpperLimitDampingUnits=N*m/(deg/s)  UpperLimitTransitionRegionWidth=0.1  UpperLimitTransitionRegionWidthUnits=deg  PositionTargetSpecify=off  PositionTargetPriority=High  PositionTargetValue=0  PositionTargetValueUnits=deg  VelocityTargetSpecify=off  VelocityTargetPriority=High  VelocityTargetValue=0  VelocityTargetValueUnits=deg/s
  Revolute Joint2 : sm_lib/Joints/Revolute Joint  JointMode=Normal  SenseConstraintForce=off  SenseConstraintForceX=off  SenseConstraintForceY=off  SenseConstraintForceZ=off  SenseConstraintTorque=off  SenseConstraintTorqueX=off  SenseConstraintTorqueY=off  SenseConstraintTorqueZ=off  SenseTotalForce=off  SenseTotalForceX=off  SenseTotalForceY=off  SenseTotalForceZ=off  SenseTotalTorque=off  SenseTotalTorqueX=off  SenseTotalTorqueY=off  SenseTotalTorqueZ=off  CompositeWrenchDir=FollowerOnBase  CompositeWrenchFrame=BaseFrame  EquilibriumPosition=0  EquilibriumPositionUnits=deg  SpringStiffness=0  SpringStiffnessUnits=N*m/deg  DampingCoefficient=0  DampingCoefficientUnits=N*m/(deg/s)  TorqueActuationMode=ComputedTorque  MotionActuationMode=InputMotion  SensePosition=on  SenseVelocity=on  SenseAcceleration=on  SenseTorqueForce=off  SenseLowerLimitTorqueForce=off  SenseUpperLimitTorqueForce=off  LowerLimitSpecify=off  LowerLimitBound=-90  LowerLimitBoundUnits=deg  LowerLimitStiffness=1e4  LowerLimitStiffnessUnits=N*m/deg  LowerLimitDamping=10  LowerLimitDampingUnits=N*m/(deg/s)  LowerLimitTransitionRegionWidth=0.1  LowerLimitTransitionRegionWidthUnits=deg  UpperLimitSpecify=off  UpperLimitBound=90  UpperLimitBoundUnits=deg  UpperLimitStiffness=1e4  UpperLimitStiffnessUnits=N*m/deg  UpperLimitDamping=10  UpperLimitDampingUnits=N*m/(deg/s)  UpperLimitTransitionRegionWidth=0.1  UpperLimitTransitionRegionWidthUnits=deg  PositionTargetSpecify=off  PositionTargetPriority=High  PositionTargetValue=0  PositionTargetValueUnits=deg  VelocityTargetSpecify=off  VelocityTargetPriority=High  VelocityTargetValue=0  VelocityTargetValueUnits=deg/s
  Revolute Joint3 : sm_lib/Joints/Revolute Joint  JointMode=Normal  SenseConstraintForce=off  SenseConstraintForceX=off  SenseConstraintForceY=off  SenseConstraintForceZ=off  SenseConstraintTorque=off  SenseConstraintTorqueX=off  SenseConstraintTorqueY=off  SenseConstraintTorqueZ=off  SenseTotalForce=off  SenseTotalForceX=off  SenseTotalForceY=off  SenseTotalForceZ=off  SenseTotalTorque=off  SenseTotalTorqueX=off  SenseTotalTorqueY=off  SenseTotalTorqueZ=off  CompositeWrenchDir=FollowerOnBase  CompositeWrenchFrame=BaseFrame  EquilibriumPosition=0  EquilibriumPositionUnits=deg  SpringStiffness=0  SpringStiffnessUnits=N*m/deg  DampingCoefficient=0  DampingCoefficientUnits=N*m/(deg/s)  TorqueActuationMode=ComputedTorque  MotionActuationMode=InputMotion  SensePosition=on  SenseVelocity=on  SenseAcceleration=on  SenseTorqueForce=off  SenseLowerLimitTorqueForce=off  SenseUpperLimitTorqueForce=off  LowerLimitSpecify=off  LowerLimitBound=-90  LowerLimitBoundUnits=deg  LowerLimitStiffness=1e4  LowerLimitStiffnessUnits=N*m/deg  LowerLimitDamping=10  LowerLimitDampingUnits=N*m/(deg/s)  LowerLimitTransitionRegionWidth=0.1  LowerLimitTransitionRegionWidthUnits=deg  UpperLimitSpecify=off  UpperLimitBound=90  UpperLimitBoundUnits=deg  UpperLimitStiffness=1e4  UpperLimitStiffnessUnits=N*m/deg  UpperLimitDamping=10  UpperLimitDampingUnits=N*m/(deg/s)  UpperLimitTransitionRegionWidth=0.1  UpperLimitTransitionRegionWidthUnits=deg  PositionTargetSpecify=on  PositionTargetPriority=High  PositionTargetValue=0  PositionTargetValueUnits=deg  VelocityTargetSpecify=off  VelocityTargetPriority=High  VelocityTargetValue=0  VelocityTargetValueUnits=deg/s
  Revolute Joint4 : sm_lib/Joints/Revolute Joint  JointMode=Normal  SenseConstraintForce=off  SenseConstraintForceX=off  SenseConstraintForceY=off  SenseConstraintForceZ=off  SenseConstraintTorque=off  SenseConstraintTorqueX=off  SenseConstraintTorqueY=off  SenseConstraintTorqueZ=off  SenseTotalForce=off  SenseTotalForceX=off  SenseTotalForceY=off  SenseTotalForceZ=off  SenseTotalTorque=off  SenseTotalTorqueX=off  SenseTotalTorqueY=off  SenseTotalTorqueZ=off  CompositeWrenchDir=FollowerOnBase  CompositeWrenchFrame=BaseFrame  EquilibriumPosition=0  EquilibriumPositionUnits=deg  SpringStiffness=0  SpringStiffnessUnits=N*m/deg  DampingCoefficient=0  DampingCoefficientUnits=N*m/(deg/s)  TorqueActuationMode=ComputedTorque  MotionActuationMode=InputMotion  SensePosition=on  SenseVelocity=on  SenseAcceleration=on  SenseTorqueForce=off  SenseLowerLimitTorqueForce=off  SenseUpperLimitTorqueForce=off  LowerLimitSpecify=off  LowerLimitBound=-90  LowerLimitBoundUnits=deg  LowerLimitStiffness=1e4  LowerLimitStiffnessUnits=N*m/deg  LowerLimitDamping=10  LowerLimitDampingUnits=N*m/(deg/s)  LowerLimitTransitionRegionWidth=0.1  LowerLimitTransitionRegionWidthUnits=deg  UpperLimitSpecify=off  UpperLimitBound=90  UpperLimitBoundUnits=deg  UpperLimitStiffness=1e4  UpperLimitStiffnessUnits=N*m/deg  UpperLimitDamping=10  UpperLimitDampingUnits=N*m/(deg/s)  UpperLimitTransitionRegionWidth=0.1  UpperLimitTransitionRegionWidthUnits=deg  PositionTargetSpecify=on  PositionTargetPriority=High  PositionTargetValue=0  PositionTargetValueUnits=deg  VelocityTargetSpecify=off  VelocityTargetPriority=High  VelocityTargetValue=0  VelocityTargetValueUnits=deg/s
  To Workspace : ToWorkspace  VariableName=r0  SaveFormat=Timeseries  SampleTime=-1
  To Workspace1 : ToWorkspace  VariableName=r0_dot  SaveFormat=Timeseries  SampleTime=-1
  To Workspace10 : ToWorkspace  VariableName=r3_dot  SaveFormat=Timeseries  SampleTime=-1
  To Workspace11 : ToWorkspace  VariableName=r3_ddot  SaveFormat=Timeseries  SampleTime=-1
  To Workspace12 : ToWorkspace  VariableName=r4_dot  SaveFormat=Timeseries  SampleTime=-1
  To Workspace13 : ToWorkspace  VariableName=r4_ddot  SaveFormat=Timeseries  SampleTime=-1
  To Workspace14 : ToWorkspace  VariableName=r4  SaveFormat=Timeseries  SampleTime=-1
  To Workspace15 : ToWorkspace  VariableName=t0_dot  SaveFormat=Timeseries  SampleTime=-1
  To Workspace16 : ToWorkspace  VariableName=t0_ddot  SaveFormat=Timeseries  SampleTime=-1
  To Workspace17 : ToWorkspace  VariableName=t0  SaveFormat=Timeseries  SampleTime=-1
  To Workspace2 : ToWorkspace  VariableName=r0_ddot  SaveFormat=Timeseries  SampleTime=-1
  To Workspace3 : ToWorkspace  VariableName=r1  SaveFormat=Timeseries  SampleTime=-1
  To Workspace4 : ToWorkspace  VariableName=r1_dot  SaveFormat=Timeseries  SampleTime=-1
  To Workspace5 : ToWorkspace  VariableName=r1_ddot  SaveFormat=Timeseries  SampleTime=-1
  To Workspace6 : ToWorkspace  VariableName=r2  SaveFormat=Timeseries  SampleTime=-1
  To Workspace7 : ToWorkspace  VariableName=r2_dot  SaveFormat=Timeseries  SampleTime=-1
  To Workspace8 : ToWorkspace  VariableName=r2_ddot  SaveFormat=Timeseries  SampleTime=-1
  To Workspace9 : ToWorkspace  VariableName=r3  SaveFormat=Timeseries  SampleTime=-1
  station : sm_lib/Body Elements/File Solid  ExtGeomFileName=.\cadModels\station.STEP  UnitType=FromFile  ExtGeomFileUnits=m  StepReaderType=HEX  ExportConvexHullGeometry=off  InertiaType=CalculateFromGeometry  Mass=1  MassUnits=kg  CenterOfMass=[0 0 0]  CenterOfMassUnits=m  MomentsOfInertia=[1 1 1]  MomentsOfInertiaUnits=kg*m^2  ProductsOfInertia=[0 0 0]  ProductsOfInertiaUnits=kg*m^2  BasedOnType=Density  Density=1000  DensityUnits=kg/m^3  DoExposeReferenceFrame=off  SerializedFrames=<Frames><Frame><Id>Frame1</Id><Value><Name>ground</Name><Origin><Source>GeometricFeature</Source><FeatureName>point 238</FeatureName></Origin><PrimaryAxis><DefinedDirection>-Z</DefinedDirection><Source>GeometricFeature</Source><SourceDirection>+Z</SourceDirection><FeatureName>segment 57</FeatureName></PrimaryAxis><SecondaryAxis><DefinedDirection>+X</DefinedDirection><Source>GeometricFeature</Source><SourceDirection>+X</SourceDirection><FeatureName>segment 59</FeatureName></SecondaryAxis></Value></Frame><Frame><Id>Frame2</Id><Value><Name>prismaticJoint</Name><Origin><Source>GeometricFeature</Source><FeatureName>circular curve 687</FeatureName></Origin><PrimaryAxis><DefinedDirection>-Z</DefinedDirection><Source>GeometricFeature</Source><SourceDirection>+Z</SourceDirection><FeatureName>circular curve 687</FeatureName></PrimaryAxis><SecondaryAxis><DefinedDirection>+X</DefinedDirection><Source>GeometricFeature</Source><SourceDirection>+X</SourceDirection><FeatureName>segment 48</FeatureName></SecondaryAxis></Value></Frame></Frames>  GraphicType=FromGeometry  MarkerShape=Sphere  MarkerSize=10  GraphicVisPropType=SimpleVisualProperties  GraphicDiffuseColor=[0.5 0.5 0.5]  GraphicSpecularColor=[0.5 0.5 0.5 1.0]  GraphicAmbientColor=[0.15 0.15 0.15 1.0]  GraphicEmissiveColor=[0.0 0.0 0.0 1.0]  GraphicShininess=75  GraphicOpacity=1.0
  output1 : PMIOPort  Side=Left
  output2 : PMIOPort  Port=2  Side=Left
  output3 : PMIOPort  Port=3  Side=Left
  output4 : PMIOPort  Port=4  Side=Left
  output5 : PMIOPort  Port=5  Side=Left
  output6 : PMIOPort  Port=6  Side=Left
  t1 : Outport
  r1 : Outport  Port=2
  r2 : Outport  Port=3
  r3 : Outport  Port=4
  r4 : Outport  Port=5
  r5 : Outport  Port=6
  wires:
  PS-Simulink Converter16/1 -> To Workspace15/1
  PS-Simulink Converter12/1 -> To Workspace10/1
  PS-Simulink Converter17/1 -> To Workspace16/1
  PS-Simulink Converter14/1 -> To Workspace12/1
  PS-Simulink Converter8/1 -> To Workspace8/1
  PS-Simulink Converter15/1 -> To Workspace13/1
  PS-Simulink Converter13/1 -> To Workspace11/1
  PS-Simulink Converter9/1 -> To Workspace4/1
  PS-Simulink Converter6/1 -> To Workspace1/1
  PS-Simulink Converter10/1 -> To Workspace5/1
  PS-Simulink Converter11/1 -> To Workspace7/1
  PS-Simulink Converter7/1 -> To Workspace2/1
  PS-Simulink Converter5/1 -> To Workspace14/1, r5/1
  PS-Simulink Converter1/1 -> To Workspace/1, r1/1
  PS-Simulink Converter/1 -> To Workspace17/1, t1/1
  PS-Simulink Converter3/1 -> To Workspace6/1, r3/1
  PS-Simulink Converter4/1 -> To Workspace9/1, r4/1
  PS-Simulink Converter2/1 -> To Workspace3/1, r2/1
  connections:
  Prismatic Joint/RConn4 -- PS-Simulink Converter17/LConn1
  Prismatic Joint/RConn3 -- PS-Simulink Converter16/LConn1
  Configuration Setup/RConn1 -- station/LConn1
  Revolute Joint4/RConn4 -- PS-Simulink Converter15/LConn1
  Revolute Joint4/RConn3 -- PS-Simulink Converter14/LConn1
  output4/RConn1 -- Revolute Joint2/LConn2
  Link5/RConn1 -- Revolute Joint4/LConn1
  Revolute Joint1/RConn3 -- PS-Simulink Converter9/LConn1
  Revolute Joint3/RConn3 -- PS-Simulink Converter12/LConn1
  Revolute Joint3/RConn4 -- PS-Simulink Converter13/LConn1
  Revolute Joint4/RConn1 -- Link6/LConn1
  Link1/RConn1 -- Revolute Joint/LConn1
  Revolute Joint3/RConn2 -- PS-Simulink Converter4/LConn1
  Revolute Joint2/RConn4 -- PS-Simulink Converter8/LConn1
  Revolute Joint1/RConn4 -- PS-Simulink Converter10/LConn1
  Revolute Joint2/RConn3 -- PS-Simulink Converter11/LConn1
  Revolute Joint4/RConn2 -- PS-Simulink Converter5/LConn1
  Revolute Joint/RConn4 -- PS-Simulink Converter7/LConn1
  output2/RConn1 -- Revolute Joint/LConn2
  Revolute Joint/RConn3 -- PS-Simulink Converter6/LConn1
  output1/RConn1 -- Prismatic Joint/LConn2
  Prismatic Joint/RConn1 -- Link1/LConn1
  Revolute Joint2/RConn2 -- PS-Simulink Converter3/LConn1
  Revolute Joint2/RConn1 -- Link4/LConn1
  Revolute Joint1/RConn2 -- PS-Simulink Converter2/LConn1
  output6/RConn1 -- Revolute Joint4/LConn2
  Link6/RConn1 -- Graphic/RConn1
  Revolute Joint/RConn2 -- PS-Simulink Converter1/LConn1
  Prismatic Joint/RConn2 -- PS-Simulink Converter/LConn1
  Revolute Joint3/RConn1 -- Link5/LConn1
  output5/RConn1 -- Revolute Joint3/LConn2
  Link2/RConn1 -- Revolute Joint1/LConn1
  Link4/RConn1 -- Revolute Joint3/LConn1
  station/RConn1 -- Prismatic Joint/LConn1
  Link3/RConn1 -- Revolute Joint2/LConn1
  Revolute Joint1/RConn1 -- Link3/LConn1
  Revolute Joint/RConn1 -- Link2/LConn1
  output3/RConn1 -- Revolute Joint1/LConn2

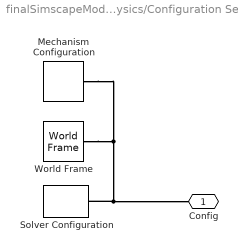
== system finalSimscapeModel/Simscape Multibody Physics/Configuration Setup ==
  Mechanism Configuration : sm_lib/Utilities/Mechanism Configuration  UniformGravity=Constant  GravityVector=[0 0 -9.80665]  GravityUnits=m/s^2  LinearizationDelta=0.001  JointModeTransitionNonlinearIterations=2
  Solver Configuration : nesl_utility/Solver Configuration  PhysicalDomain=network_engine_domain  SubClassName=solver  LeftPortType=input  RightPortType=generic  Tones=[]  Harmonics=[]  SimulateNoise=off  Profile=off  UseLocalSampling=off  EnableSwitchedLinearOptims=on  FrequencyDomain=off  UseCCode=off  RelTol=0.001  AbsTol=1e-06  MinStep=1e-09  ToWorkspace=off  RevertToSquareIcSolve=off  NumHomotopyIterations=100  PhasorMode=off  PhasorModeNumHarmonics=1  DoDC=off  ResidualTolerance=1e-09  UseLocalSolver=off  LocalSolverChoice=NE_BACKWARD_EULER_ADVANCER  LocalSolverSampleTime=0.001  DoFixedCost=off  MaxNonlinIter=3  MaxModeIter=2  ComputeImpulses=off  ImpulseIterations=2  LinearAlgebra=auto  EquationFormulation=NE_TIME_EF  DelaysMemoryBudget=1024  AutomaticFiltering=on  FilteringTimeConstant=0.001  PartitionStorageMethod=AS_NEEDED  PartitionMemoryBudget=1024  PartitionMethod=ROBUST
      settings: SourceProductBaseCode=PW,SS
  World Frame : sm_lib/Frames and Transforms/World Frame
  Config : PMIOPort  Side=Right
  connections:
  Mechanism Configuration/RConn1 -- Config/RConn1 -- Solver Configuration/RConn1 -- World Frame/RConn1

== matlab function finalSimscapeModel/MATLAB 3D Simuluation/states ==
  data: t1 input; v1 output; r1 input; r2 input; r3 input; r4 input; r5 input; v2 output; v3 output; v4 output; v5 output; v6 output
function [v1,v2,v3,v4,v5,v6] = fcn(t1,r1,r2,r3,r4,r5)
v1 = [0 0 -t1];
v2 = [0 0 -1 r1];
v3 = [0 0 -1 r2];
v4 = [1 0 0 r3];
v5 = [0.16232 0.077123 0.98372 -r4];
v6 = [1 0 0 r5];

== matlab function finalSimscapeModel/MATLAB Function ==
  data: a input; y output; b input
function y = fcn(a,b)
    if a < b || a > 30+b
        y = true;
    else
        y = false;
    end
end
